simulink model "color_image"  (R2022a)
settings: Solver=VariableStepAuto  StartTime=0.0  StopTime=10.0  RelTol=1e-3
libraries: simulink x6, parrotlib x1
settings Model: Creator=sjoer  LastModifiedBy=sjoer

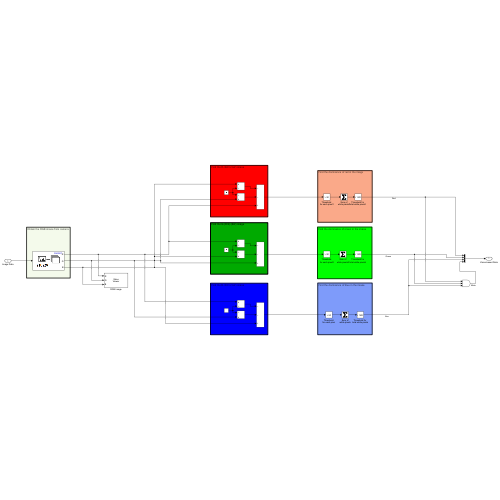
[thumbnail: Simulink's stored preview of the top-level diagram]
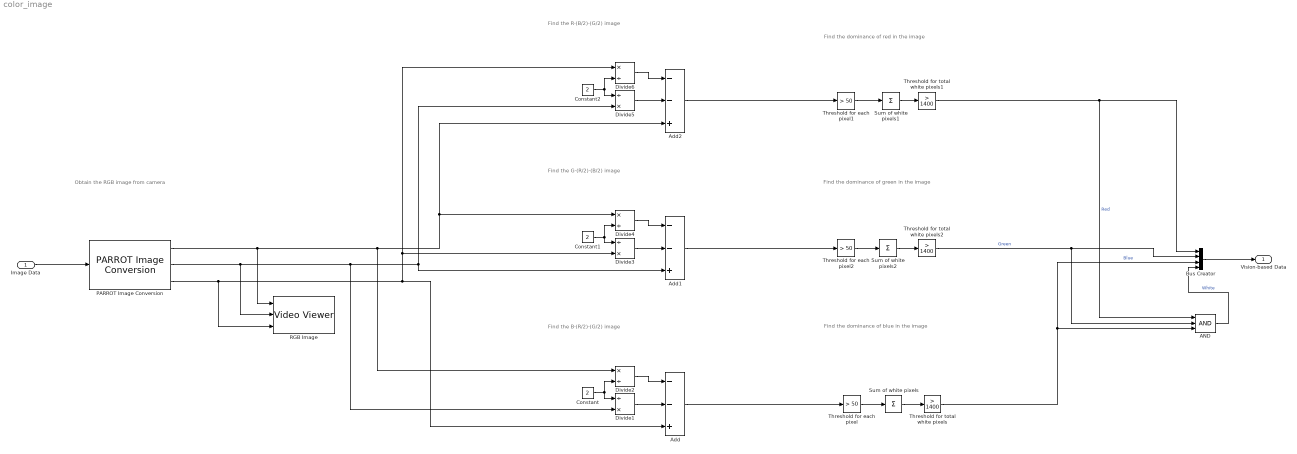
== system color_image ==
  note: Find the dominance of blue in the image
  note: Find the G-(R/2)-(B/2) image
  note: Obtain the RGB image from camera
  note: Find the B-(R/2)-(G/2) image
  note: Find the dominance of green in the image
  note: Find the dominance of red in the image
  note: Find the R-(B/2)-(G/2) image
  Image Data : Inport
  AND : Logic  Inputs=3  IconShape=distinctive  AllPortsSameDT=off  OutDataTypeStr=boolean
  Add : Sum  Inputs=--+
  Add1 : Sum  Inputs=--+
  Add2 : Sum  Inputs=--+
  Bus Creator : BusCreator  Inputs=4
  Constant : Constant  Value=2
  Constant1 : Constant  Value=2
  Constant2 : Constant  Value=2
  Divide1 : Product  Inputs=/*
  Divide2 : Product  Inputs=*/
  Divide3 : Product  Inputs=/*
  Divide4 : Product  Inputs=*/
  Divide5 : Product  Inputs=/*
  Divide6 : Product  Inputs=*/
  PARROT Image Conversion : parrotlib/PARROT Image Conversion  ImageFormat=RGB  R=on  Y=on  G=on  U=on  B=on  V=on
  RGB Image : VideoViewer  imagePorts=separate color signals  FigPos=[1088 996 418 304]
  Sum of white pixels : Sum  Inputs=+  OutDataTypeStr=uint16
  Sum of white pixels1 : Sum  Inputs=+  OutDataTypeStr=uint16
  Sum of white pixels2 : Sum  Inputs=+  OutDataTypeStr=uint16
  Threshold for each pixel : simulink/Logic and Bit Operations/Compare To Constant  relop=>  const=50  OutDataTypeStr=boolean
  Threshold for each pixel1 : simulink/Logic and Bit Operations/Compare To Constant  relop=>  const=50  OutDataTypeStr=boolean
  Threshold for each pixel2 : simulink/Logic and Bit Operations/Compare To Constant  relop=>  const=50  OutDataTypeStr=boolean
  Threshold for total white pixels : simulink/Logic and Bit Operations/Compare To Constant  relop=>  const=1400  OutDataTypeStr=boolean
  Threshold for total white pixels1 : simulink/Logic and Bit Operations/Compare To Constant  relop=>  const=1400  OutDataTypeStr=boolean
  Threshold for total white pixels2 : simulink/Logic and Bit Operations/Compare To Constant  relop=>  const=1400  OutDataTypeStr=boolean
  Vision-based Data : Outport  VectorParamsAs1DForOutWhenUnconnected=off
  wires:
  PARROT Image Conversion/3 -> RGB Image/3, Divide3/2, Divide6/1, Add/3
  Divide4/1 -> Add1/1
  Constant1/1 -> Divide3/1, Divide4/2
  Image Data/1 -> PARROT Image Conversion/1
  Sum of white pixels/1 -> Threshold for total white pixels/1
  Divide2/1 -> Add/1
  Add/1 -> Threshold for each pixel/1
  Constant/1 -> Divide1/1, Divide2/2
  Bus Creator/1 -> Vision-based Data/1
  Add1/1 -> Threshold for each pixel2/1
  Add2/1 -> Threshold for each pixel1/1
  PARROT Image Conversion/2 -> RGB Image/2, Divide1/2, Divide5/2, Add1/3
  Sum of white pixels2/1 -> Threshold for total white pixels2/1
  Threshold for each pixel/1 -> Sum of white pixels/1
  Threshold for each pixel2/1 -> Sum of white pixels2/1
  Threshold for total white pixels2/1 -> AND/2, Bus Creator/2  "Green"
  Divide3/1 -> Add1/2
  Threshold for each pixel1/1 -> Sum of white pixels1/1
  Sum of white pixels1/1 -> Threshold for total white pixels1/1
  Divide1/1 -> Add/2
  Divide5/1 -> Add2/2
  Divide6/1 -> Add2/1
  Constant2/1 -> Divide5/1, Divide6/2
  PARROT Image Conversion/1 -> RGB Image/1, Divide2/1, Divide4/1, Add2/3
  Threshold for total white pixels/1 -> AND/3, Bus Creator/3  "Blue"
  Threshold for total white pixels1/1 -> AND/1, Bus Creator/1  "Red"
  AND/1 -> Bus Creator/4  "White"
